simulink model "quadrotor_model+planing"  (R2021a)
settings: Solver=VariableStepAuto  StartTime=0.0  StopTime=inf  RelTol=1e-3
libraries: simulink x1
settings Model: EnablePacing=on  Creator=amejiyopakapak  LastModifiedBy=user

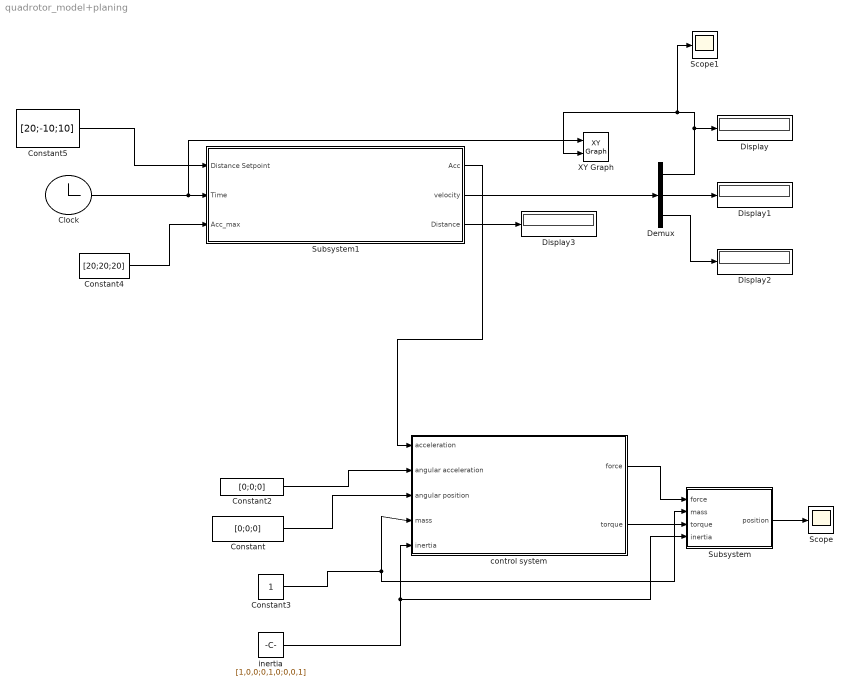
== system quadrotor_model+planing ==
  Clock : Clock
  Constant : Constant  Value=[0;0;0]  VectorParams1D=off
  Constant2 : Constant  Value=[0;0;0]  VectorParams1D=off
  Constant3 : Constant
  Constant4 : Constant  Value=[20;20;20]
  Constant5 : Constant  Value=[20;-10;10]
  Demux : Demux  Outputs=3
  Display{,1..3} (4 alike) : Display
  Scope : Scope
  Scope1 : Scope
  Subsystem : Subsystem
  Subsystem1 : Subsystem
  XY Graph : simulink/Sinks/XY Graph  xmin=-100  xmax=100  ymin=-100  ymax=100  st=-1
  control system : Subsystem
  inertia : Constant  Value=[1,0,0;0,1,0;0,0,1]  VectorParams1D=off
  wires:
  Constant/1 -> control system/3(angular position)
  Constant2/1 -> control system/2(angular acceleration)
  Constant3/1 -> control system/4(mass), Subsystem/2(mass)
  inertia/1 -> Subsystem/4(inertia), control system/5(inertia)
  control system/1(force) -> Subsystem/1(force)
  control system/2(torque) -> Subsystem/3(torque)
  Subsystem/1(position) -> Scope/1
  Demux/3 -> Display2/1
  Subsystem1/2(velocity) -> Demux/1
  Clock/1 -> XY Graph/1, Subsystem1/2(Time)
  Demux/2 -> Display1/1
  Constant4/1 -> Subsystem1/3(Acc_max)
  Demux/1 -> Scope1/1, XY Graph/2, Display/1
  Constant5/1 -> Subsystem1/1(Distance Setpoint)
  Subsystem1/3(Distance) -> Display3/1
  Subsystem1/1("Acc ") -> control system/1(acceleration)

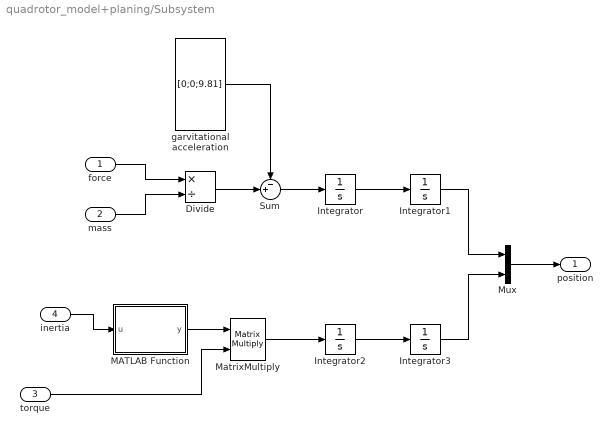
== system quadrotor_model+planing/Subsystem ==
  force : Inport
  mass : Inport  Port=2
  torque : Inport  Port=3
  inertia : Inport  Port=4
  Divide : Product  Inputs=*/
  Integrator{,1..3} (4 alike) : Integrator
  MATLAB Function : MATLAB Function  TreatAsAtomicUnit=on
  MatrixMultiply : Product  Multiplication=Matrix(*)
  Mux : Mux  Inputs=2
  Sum : Sum  Inputs=-+|
  garvitational acceleration : Constant  Value=[0;0;9.81]  VectorParams1D=off
  position : Outport
  wires:
  Mux/1 -> position/1
  garvitational acceleration/1 -> Sum/1
  MatrixMultiply/1 -> Integrator2/1
  MATLAB Function/1(y) -> MatrixMultiply/1
  torque/1 -> MatrixMultiply/2
  Sum/1 -> Integrator/1
  Integrator1/1 -> Mux/1
  Divide/1 -> Sum/2
  Integrator2/1 -> Integrator3/1
  Integrator3/1 -> Mux/2
  force/1 -> Divide/1
  mass/1 -> Divide/2
  inertia/1 -> MATLAB Function/1(u)
  Integrator/1 -> Integrator1/1

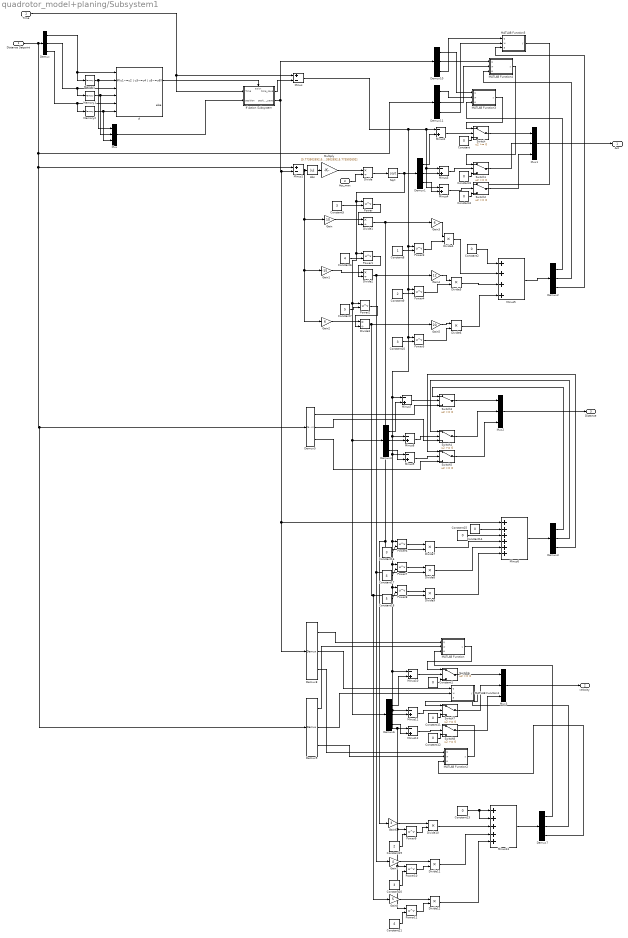
== system quadrotor_model+planing/Subsystem1 ==
  Distance Setpoint : Inport
  Time : Inport  Port=2
  Acc_max : Inport  Port=3
  Abs : Abs
  Constant{,1..4,11..15} (10 alike) : Constant  Value=0
  Constant{5,10,16,20} (4 alike) : Constant  Value=3
  Constant17 : Constant  Value=4
  Constant18 : Constant  Value=5
  Constant19 : Constant  Value=2
  Constant21 : Constant  Value=4
  Constant6 : Constant  Value=4
  Constant7 : Constant  Value=5
  Constant8 : Constant
  Constant9 : Constant  Value=2
  Demux{,1..11} (12 alike) : Demux  Outputs=3
  Divide{,1..3} (4 alike) : Product  Inputs=*/
  Divide{4..12} (9 alike) : Product  Inputs=**
  Gain : Gain  Gain=10
  Gain1 : Gain  Gain=-15
  Gain2 : Gain  Gain=6
  Gain3 : Gain  Gain=6
  Gain4 : Gain  Gain=12
  Gain5 : Gain  Gain=20
  Gain6 : Gain  Gain=3
  Gain7 : Gain  Gain=4
  Gain8 : Gain  Gain=5
  If : If  NumInputs=6  IfExpression=(u1~=u2 | u3~=u4 | u5~=u6)
  If Action Subsystem : Subsystem  TreatAsAtomicUnit=on
  MATLAB Function : MATLAB Function  TreatAsAtomicUnit=on
  MATLAB Function1 : MATLAB Function  TreatAsAtomicUnit=on
  MATLAB Function2 : MATLAB Function  TreatAsAtomicUnit=on
  MATLAB Function3 : MATLAB Function  TreatAsAtomicUnit=on
  MATLAB Function4 : MATLAB Function  TreatAsAtomicUnit=on
  MATLAB Function5 : MATLAB Function  TreatAsAtomicUnit=on
  Memory : Memory
  Memory1 : Memory
  Memory2 : Memory
  Minus : Sum  Inputs=+-
  Minus1 : Sum  Inputs=+-
  Minus{2..4,7..12} (9 alike) : Sum  Inputs=-+
  Minus13 : Sum  Inputs=+++++
  Minus5 : Sum  Inputs=++++
  Minus6 : Sum  Inputs=++++++
  Multiply : Gain  Gain=[5.773502692;5.773502692;5.773502692]
  Mux{,1..3} (4 alike) : Mux  Inputs=3
  Power{,1..11} (12 alike) : Math  Operator=pow  SaturateOnIntegerOverflow=on
  Sqrt : Sqrt  SaturateOnIntegerOverflow=on
  Switch{,1..8} (9 alike) : Switch
  "Acc " : Outport
  velocity : Outport  Port=2
  Distance : Outport  Port=3
  wires:
  If/1 -> If Action Subsystem/Action
  Memory/1 -> Mux/1, If/2
  Time/1 -> Minus/1, If Action Subsystem/1(Time)
  Demux/1 -> Memory/1, If/1
  Memory1/1 -> Mux/2, If/4
  Memory2/1 -> Mux/3, If/6
  Demux/2 -> Memory1/1, If/3
  Demux/3 -> Memory2/1, If/5
  Mux/1 -> If Action Subsystem/2(position)
  Multiply/1 -> Divide/1
  Acc_max/1 -> Divide/2
  Divide/1 -> Sqrt/1
  Constant/1 -> Switch/3
  Mux1/1 -> "Acc "/1
  Switch/1 -> Mux1/1
  Constant3/1 -> Switch1/3
  Constant4/1 -> Switch2/3
  Switch1/1 -> Mux1/2
  Switch2/1 -> Mux1/3
  Demux1/2 -> Minus3/2
  Minus3/1 -> Switch1/2
  Demux1/3 -> Minus4/2
  Minus4/1 -> Switch2/2
  Gain/1 -> Divide1/1
  Constant5/1 -> Power/2
  Power/1 -> Divide1/2
  Constant6/1 -> Power1/2
  Gain1/1 -> Divide2/1
  Power1/1 -> Divide2/2
  Constant7/1 -> Power2/2
  Demux1/1 -> Minus2/2
  Minus1/1 -> Gain1/1, Gain2/1, Gain/1, Abs/1
  Power2/1 -> Divide3/2
  Gain2/1 -> Divide3/1
  Minus5/1 -> Demux2/1
  Demux2/1 -> MATLAB Function3/3(e)
  Demux2/3 -> MATLAB Function5/3(e)
  Constant2/1 -> Minus5/1
  Gain3/1 -> Divide4/1
  Divide4/1 -> Minus5/2
  Gain4/1 -> Divide5/1
  Divide5/1 -> Minus5/3
  Gain5/1 -> Divide6/1
  Divide6/1 -> Minus5/4
  Power3/1 -> Divide4/2
  Constant8/1 -> Power3/2
  Constant9/1 -> Power4/2
  Constant10/1 -> Power5/2
  Minus2/1 -> Switch/2
  Power4/1 -> Divide5/2
  Power5/1 -> Divide6/2
  Switch5/1 -> Mux2/3
  Minus7/1 -> Switch3/2
  Demux4/1 -> Minus7/2
  Demux4/3 -> Minus9/2
  Demux3/3 -> Switch5/1
  Switch3/1 -> Mux2/1
  Demux3/2 -> Switch4/1
  Demux3/1 -> Switch3/1
  Minus9/1 -> Switch5/2
  Minus8/1 -> Switch4/2
  Demux4/2 -> Minus8/2
  Switch4/1 -> Mux2/2
  Demux5/3 -> Switch5/3
  Demux5/1 -> Switch3/3
  Demux5/2 -> Switch4/3
  Mux2/1 -> Distance/1
  Minus6/1 -> Demux3/1
  If Action Subsystem/2(position_save) -> Demux8/1, Minus6/1, Minus1/2, Demux10/1
  Constant14/1 -> Minus6/2
  Constant15/1 -> Minus6/3
  Divide7/1 -> Minus6/4
  Divide8/1 -> Minus6/5
  Divide9/1 -> Minus6/6
  Power6/1 -> Divide7/1
  Power7/1 -> Divide8/1
  Power8/1 -> Divide9/1
  Constant16/1 -> Power6/2
  Constant17/1 -> Power7/2
  Constant18/1 -> Power8/2
  Distance Setpoint/1 -> Demux9/1, Demux5/1, Minus1/1, Demux11/1, Demux/1
  Abs/1 -> Multiply/1
  Switch8/1 -> Mux3/3
  Minus10/1 -> Switch6/2
  Sqrt/1 -> Demux4/1, Demux6/1, Power2/1, Power1/1, Power/1, Demux1/1
  Demux6/1 -> Minus10/2
  Demux6/3 -> Minus12/2
  Demux7/3 -> MATLAB Function2/3(e)
  Switch6/1 -> Mux3/1
  Demux7/2 -> MATLAB Function1/3(e)
  Demux7/1 -> MATLAB Function/3(e)
  Minus/1 -> Minus4/1, Minus3/1, Minus2/1, Power3/1, Minus7/1, Power6/1, Minus10/1, Minus11/1, Power9/1, Power11/1, Power10/1, Minus12/1, Power8/1, Power7/1, Minus9/1, Minus8/1, Power5/1, Power4/1
  Minus12/1 -> Switch8/2
  Minus11/1 -> Switch7/2
  Demux6/2 -> Minus11/2
  Switch7/1 -> Mux3/2
  Constant12/1 -> Switch8/3
  Constant1/1 -> Switch6/3
  Constant11/1 -> Switch7/3
  Mux3/1 -> velocity/1
  Minus13/1 -> Demux7/1
  Constant13/1 -> Minus13/2, Minus13/1
  Divide10/1 -> Minus13/3
  Divide11/1 -> Minus13/4
  Divide12/1 -> Minus13/5
  Gain6/1 -> Divide10/1
  Gain7/1 -> Divide11/1
  Gain8/1 -> Divide12/1
  Divide1/1 -> Gain3/1, Gain6/1, Divide7/2
  Divide2/1 -> Gain4/1, Gain7/1, Divide8/2
  Divide3/1 -> Gain5/1, Gain8/1, Divide9/2
  Power9/1 -> Divide10/2
  Power11/1 -> Divide12/2
  Power10/1 -> Divide11/2
  Constant19/1 -> Power9/2
  Constant20/1 -> Power10/2
  Constant21/1 -> Power11/2
  Demux8/1 -> MATLAB Function/1(q)
  Demux9/1 -> MATLAB Function/2(w)
  MATLAB Function/1(y) -> Switch6/1
  Demux8/2 -> MATLAB Function1/1(q)
  Demux9/2 -> MATLAB Function1/2(w)
  MATLAB Function1/1(y) -> Switch7/1
  Demux8/3 -> MATLAB Function2/1(q)
  Demux9/3 -> MATLAB Function2/2(w)
  MATLAB Function2/1(y) -> Switch8/1
  Demux10/1 -> MATLAB Function3/1(q)
  Demux11/1 -> MATLAB Function3/2(w)
  Demux10/2 -> MATLAB Function4/1(q)
  Demux11/2 -> MATLAB Function4/2(w)
  Demux2/2 -> MATLAB Function4/3(e)
  MATLAB Function4/1(y) -> Switch1/1
  Demux11/3 -> MATLAB Function5/2(w)
  Demux10/3 -> MATLAB Function5/1(q)
  MATLAB Function5/1(y) -> Switch2/1
  If Action Subsystem/1("time_save ") -> Minus/2
  MATLAB Function3/1(y) -> Switch/1

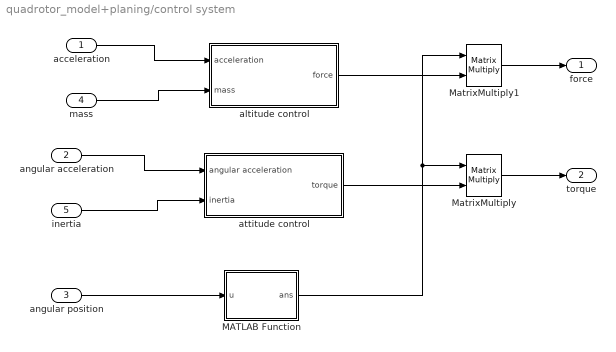
== system quadrotor_model+planing/control system ==
  acceleration : Inport
  angular acceleration : Inport  Port=2
  angular position : Inport  Port=3
  mass : Inport  Port=4
  inertia : Inport  Port=5
  MATLAB Function : MATLAB Function  TreatAsAtomicUnit=on
  MatrixMultiply : Product  Multiplication=Matrix(*)
  MatrixMultiply1 : Product  Multiplication=Matrix(*)
  altitude control : Subsystem
  attitude control : Subsystem
  force : Outport
  torque : Outport  Port=2
  wires:
  acceleration/1 -> altitude control/1(acceleration)
  angular acceleration/1 -> attitude control/1(angular acceleration)
  angular position/1 -> MATLAB Function/1(u)
  MATLAB Function/1(ans) -> MatrixMultiply1/1, MatrixMultiply/1
  MatrixMultiply/1 -> torque/1
  attitude control/1(torque) -> MatrixMultiply/2
  MatrixMultiply1/1 -> force/1
  altitude control/1(force) -> MatrixMultiply1/2
  inertia/1 -> attitude control/2(inertia)
  mass/1 -> altitude control/2(mass)

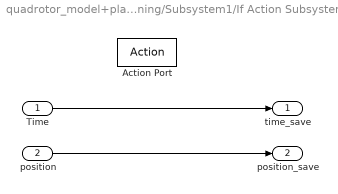
== system quadrotor_model+planing/Subsystem1/If Action Subsystem ==
  Time : Inport
  position : Inport  Port=2
  Action Port : ActionPort  InitializeStates=reset  PropagateVarSize=During execution  ActionPortLabel=if((u1~=u2 | u3~=u4 | u5~=u6))
  "time_save " : Outport
  position_save : Outport  Port=2
  wires:
  Time/1 -> "time_save "/1
  position/1 -> position_save/1

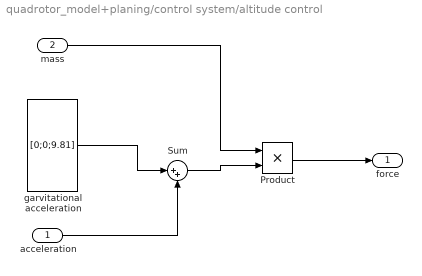
== system quadrotor_model+planing/control system/altitude control ==
  acceleration : Inport
  mass : Inport  Port=2
  Product : Product
  Sum : Sum  Inputs=|++
  garvitational acceleration : Constant  Value=[0;0;9.81]  VectorParams1D=off
  force : Outport
  wires:
  Sum/1 -> Product/2
  garvitational acceleration/1 -> Sum/1
  Product/1 -> force/1
  acceleration/1 -> Sum/2
  mass/1 -> Product/1

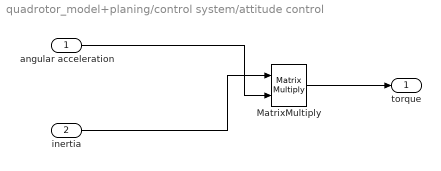
== system quadrotor_model+planing/control system/attitude control ==
  angular acceleration : Inport
  inertia : Inport  Port=2
  MatrixMultiply : Product  Multiplication=Matrix(*)
  torque : Outport
  wires:
  MatrixMultiply/1 -> torque/1
  angular acceleration/1 -> MatrixMultiply/2
  inertia/1 -> MatrixMultiply/1

== matlab function quadrotor_model+planing/control system/MATLAB Function ==
  data: u input; ans output
function ans = rotationMatrix(u)
    r = u(1);
    p = u(2);
    y = u(3);
    ans = [cos(y)*cos(r), (-sin(y)*cos(r)) + (cos(y)*sin(p)*sin(r)), sin(y)*sin(r) + cos(y)*sin(p)*cos(r);sin(y)*cos(p), cos(y)*cos(r)+sin(y)*sin(p)*sin(r), -cos(y)*sin(r) + sin(y)*sin(p)*cos(r);-sin(p),cos(p)*sin(r),cos(p)*cos(r)];
ans;

== matlab function quadrotor_model+planing/Subsystem1/MATLAB Function ==
  data: q input; y output; w input; e input
function y = fcn(q,w,e)
  if(q==w)
    y=0;
  else 
    y = e; 
  end

end

== matlab function quadrotor_model+planing/Subsystem1/MATLAB Function1 ==
  data: q input; y output; w input; e input
function y = fcn(q,w,e)
  if(q==w)
    y=0;
  else 
    y = e; 
  end

end

== matlab function quadrotor_model+planing/Subsystem1/MATLAB Function2 ==
  data: q input; y output; w input; e input
function y = fcn(q,w,e)
  if(q==w)
    y=0;
  else 
    y = e; 
  end

end

== matlab function quadrotor_model+planing/Subsystem1/MATLAB Function3 ==
  data: q input; y output; w input; e input
function y = fcn(q,w,e)
  if(q==w)
    y=0;
  else 
    y = e; 
  end

end

== matlab function quadrotor_model+planing/Subsystem1/MATLAB Function4 ==
  data: q input; y output; w input; e input
function y = fcn(q,w,e)
  if(q==w)
    y=0;
  else 
    y = e; 
  end

end

== matlab function quadrotor_model+planing/Subsystem1/MATLAB Function5 ==
  data: q input; y output; w input; e input
function y = fcn(q,w,e)
  if(q==w)
    y=0;
  else 
    y = e; 
  end

end

== matlab function quadrotor_model+planing/Subsystem/MATLAB Function ==
  data: u input; y output
function y = inverseMatrix(u)

y = inv(u);
